simulink model "sSpiegelPadStromSensor"  (R2012b)
settings: Solver=ode45  StartTime=0.0  StopTime=10.0  RelTol=1e-3
values from neighbouring files (symbols this model uses):
  J = 93.3e-9    (= 9.33e-08)    [msSpiegel.m]    (also in msSpiegel_PID.m; msSpiegel_Pad.m; msSpiegel_Pad_Neue_Werte.m = 9.33e-09; msSpiegel_Pad_Neue_Werte_Strom.m = 9.33e-10)
  KMPHI = 6.3e-2    (= 0.063)    [msSpiegel.m]    (also in msSpiegel_PID.m; msSpiegel_Pad.m; msSpiegel_Pad_Neue_Werte.m = 0.035; msSpiegel_Pad_Neue_Werte_Strom.m = 0.035)
  LA = RA*TA    (= 0.000448)    [msSpiegel.m]    (also in msSpiegel_PID.m; msSpiegel_Pad.m; msSpiegel_Pad_Neue_Werte.m = 3e-06; msSpiegel_Pad_Neue_Werte_Strom.m = 3e-06)
  Mspiegel = 130.25e-3    (= 0.13025)    [msSpiegel.m]    (also in msSpiegel_PID.m; msSpiegel_Pad.m; msSpiegel_Pad_Neue_Werte_Strom.m = 3.025e-05; msSpiegelundSensor.m = 3.025e-05)
  phi = 0.4    [Sensor_initieren.m]    (also in msSpiegel.m = 0.174532925199; msSpiegel_PID.m = 0.349065850399; msSpiegel_Pad.m = 0.349065850399; msSpiegel_Pad_Neue_Werte.m = 0.349065850399)
  r = []    [faltungsfunktionen.m]    (also in faltungsfunktionen3.m; msSpiegel.m = 6e-05; msSpiegel_PID.m = 6e-05; msSpiegel_Pad.m = 6e-05)
  RA = .16    (= 0.16)    [msSpiegel.m]    (also in msSpiegel_PID.m; msSpiegel_Pad.m; msSpiegel_Pad_Neue_Werte.m = 0.1; msSpiegel_Pad_Neue_Werte_Strom.m = 0.1)
settings Model: Creator=froriep  LastModifiedBy=michamann
settings DataIOCC: SignalLoggingSaveFormat=ModelDataLogs
settings DebuggingCC: FcnCallInpInsideContextMsg=EnableAllAsWarning
settings GRTTargetCC: CombineOutputUpdateFcns=off  GRTInterface=on

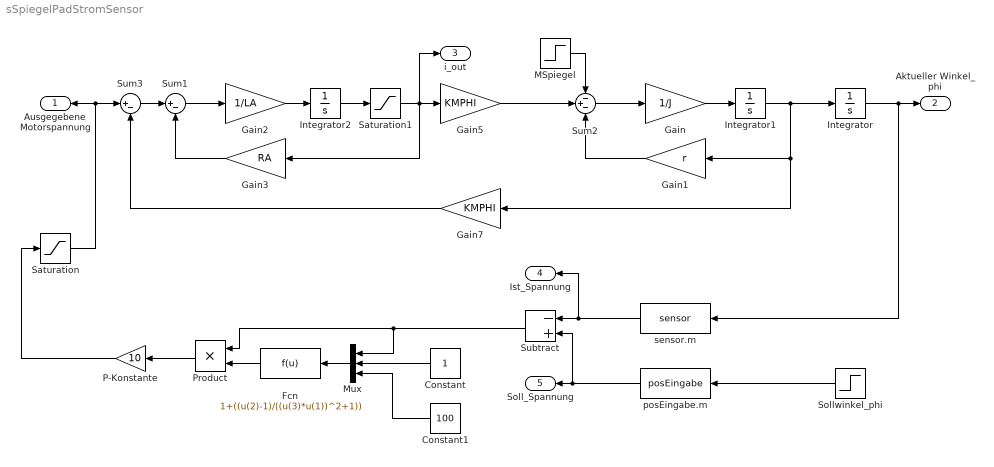
== system sSpiegelPadStromSensor ==
  Constant : Constant
  Constant1 : Constant  Value=100
  Fcn : Fcn  Expr=1+((u(2)-1)/((u(3)*u(1))^2+1))
  Gain : Gain  Gain=1/J
  Gain1 : Gain  Gain=r
  Gain2 : Gain  Gain=1/LA
  Gain3 : Gain  Gain=RA
  Gain5 : Gain  Gain=KMPHI
  Gain7 : Gain  Gain=KMPHI
  Integrator : Integrator
  Integrator1 : Integrator
  Integrator2 : Integrator
  MSpiegel : Step  Time=0  After=Mspiegel  SampleTime=0
  Mux : Mux  Inputs=3
  P-Konstante : Gain  Gain=10
  Product : Product  RndMeth=Zero
  Saturation : Saturate  UpperLimit=24  LowerLimit=-24
  Saturation1 : Saturate  UpperLimit=10  LowerLimit=-10
  Sollwinkel_phi : Step  Time=100  Before=phi  After=phi  SampleTime=0
  Subtract : Sum  Inputs=-+  AccumDataTypeStr=double  OutDataTypeStr=double
  Sum1 : Sum  Inputs=|+-
  Sum2 : Sum  Inputs=-+-
  Sum3 : Sum  Inputs=|+-
  posEingabe.m : MATLABFcn  MATLABFcn=posEingabe
  sensor.m : MATLABFcn  MATLABFcn=sensor
  "Ausgegebene Motorspannung " : Outport
  Aktueller Winkel_phi : Outport  Port=2
  i_out : Outport  Port=3
  Ist_Spannung : Outport  Port=4
  Soll_Spannung : Outport  Port=5
  wires:
  Gain/1 -> Integrator1/1
  Sum2/1 -> Gain/1
  Gain1/1 -> Sum2/3
  Gain2/1 -> Integrator2/1
  Sum1/1 -> Gain2/1
  Gain5/1 -> Sum2/2
  MSpiegel/1 -> Sum2/1
  Sum3/1 -> Sum1/1
  Gain3/1 -> Sum1/2
  Gain7/1 -> Sum3/2
  Integrator/1 -> sensor.m/1, Aktueller Winkel_phi/1
  Subtract/1 -> Product/1, Mux/1
  Product/1 -> P-Konstante/1
  Fcn/1 -> Product/2
  Mux/1 -> Fcn/1
  Constant/1 -> Mux/2
  Constant1/1 -> Mux/3
  P-Konstante/1 -> Saturation/1
  Saturation/1 -> "Ausgegebene Motorspannung "/1, Sum3/1
  Integrator2/1 -> Saturation1/1
  Saturation1/1 -> i_out/1, Gain3/1, Gain5/1
  sensor.m/1 -> Ist_Spannung/1, Subtract/1
  posEingabe.m/1 -> Soll_Spannung/1, Subtract/2
  Integrator1/1 -> Gain7/1, Gain1/1, Integrator/1
  Sollwinkel_phi/1 -> posEingabe.m/1
